simulink model "buck_convertor"  (R2015a)
settings: Solver=ode45  StartTime=0  StopTime=10.5  RelTol=1e-3
libraries: simulink x1, powerlib_meascontrol x1
settings Model: Creator=Dell  LastModifiedBy=Dell

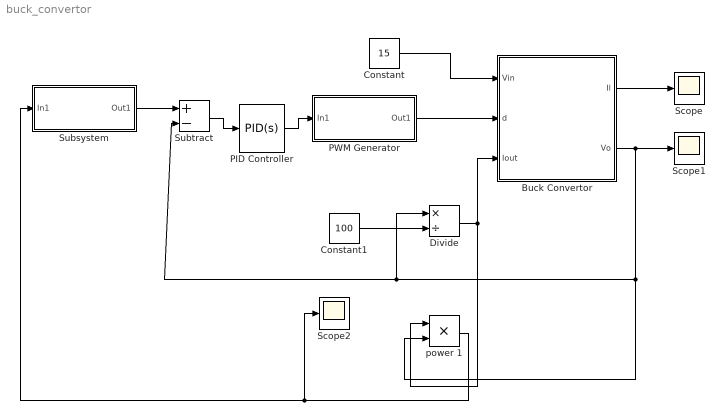
== system buck_convertor ==
  Buck Convertor : Subsystem
  Constant : Constant  Value=15
  Constant1 : Constant  Value=100
  Divide : Product  Inputs=*/
  PID Controller : simulink/Continuous/PID Controller  Controller=PID  TimeDomain=Continuous-time  SampleTime=-1  IntegratorMethod=Forward Euler  FilterMethod=Forward Euler  Form=Parallel  UseFilter=on  ControllerParametersSource=internal  P=1  I=2  D=0  N=1.2  InitialConditionSource=internal  InitialConditionForIntegrator=0  InitialConditionForFilter=0  ExternalReset=none  LimitOutput=off  UpperSaturationLimit=inf  LowerSaturationLimit=-inf  LinearizeAsGain=on  AntiWindupMode=none  Kb=1  TrackingMode=off  Kt=1  PParamMin=[]  PParamMax=[]  IParamMin=[]  IParamMax=[]  DParamMin=[]  DParamMax=[]  NParamMin=[]  NParamMax=[]  KbParamMin=[]  KbParamMax=[]  KtParamMin=[]  KtParamMax=[]  POutMin=[]  POutMax=[]  IOutMin=[]  IOutMax=[]  DOutMin=[]  DOutMax=[]  NOutMin=[]  NOutMax=[]  KbOutMin=[]  KbOutMax=[]  KtOutMin=[]  KtOutMax=[]  IntegratorOutMin=[]  IntegratorOutMax=[]  FilterOutMin=[]  FilterOutMax=[]  SumOutMin=[]  SumOutMax=[]  SumI1OutMin=[]  SumI1OutMax=[]  SumI2OutMin=[]  SumI2OutMax=[]  SumI3OutMin=[]  SumI3OutMax=[]  SumDOutMin=[]  SumDOutMax=[]  SaturationOutMin=[]  SaturationOutMax=[]  IntegratorContinuousStateAttributes=''  IntegratorStateMustResolveToSignalObject=off  IntegratorRTWStateStorageClass=Auto  FilterContinuousStateAttributes=''  FilterStateMustResolveToSignalObject=off  FilterRTWStateStorageClass=Auto  DifferentiatorICPrevScaledInput=0  DifferentiatorOutMin=[]  DifferentiatorOutMax=[]
  PWM Generator : Subsystem
  Scope : Scope
  Scope1 : Scope
      settings: YMin=16.825  YMax=17.025
  Scope2 : Scope
      settings: YMin=16.825  YMax=17.025  SaveName=ScopeData5
  Subsystem : Subsystem
  Subtract : Sum  Inputs=+-
  power 1 : Product  Inputs=**
  wires:
  Subtract/1 -> PID Controller/1
  PID Controller/1 -> PWM Generator/1(In1)
  PWM Generator/1(Out1) -> Buck Convertor/2(d)
  Divide/1 -> Buck Convertor/3(Iout), power 1/1
  Constant1/1 -> Divide/2
  Buck Convertor/1(Il) -> Scope/1
  Buck Convertor/2(Vo) -> Scope1/1, power 1/2, Divide/1, Subtract/2
  Subsystem/1(Out1) -> Subtract/1
  power 1/1 -> Scope2/1, Subsystem/1(In1)
  Constant/1 -> Buck Convertor/1(Vin)

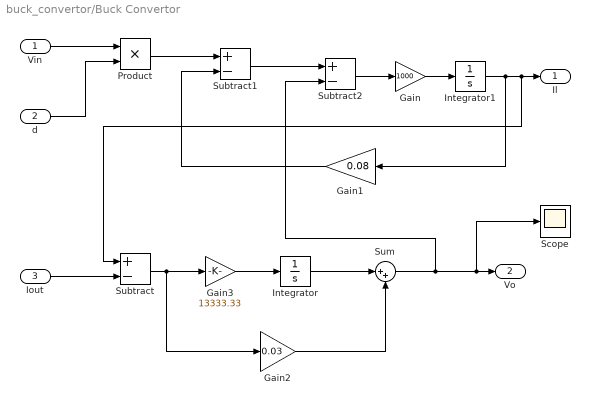
== system buck_convertor/Buck Convertor ==
  Vin : Inport
  d : Inport  Port=2
  Iout : Inport  Port=3
  Gain : Gain  Gain=1000
  Gain1 : Gain  Gain=0.08
  Gain2 : Gain  Gain=0.03
  Gain3 : Gain  Gain=13333.33
  Integrator : Integrator
  Integrator1 : Integrator
  Product : Product
  Scope : Scope
      settings: YMin=16.25  YMax=17.75  SaveName=ScopeData4
  Subtract : Sum  Inputs=+-
  Subtract1 : Sum  Inputs=+-
  Subtract2 : Sum  Inputs=+-
  Sum : Sum  Inputs=|++
  Il : Outport
  Vo : Outport  Port=2
  wires:
  Sum/1 -> Vo/1, Scope/1, Subtract2/2
  Gain2/1 -> Sum/2
  Integrator/1 -> Sum/1
  Gain3/1 -> Integrator/1
  Subtract/1 -> Gain3/1, Gain2/1
  Iout/1 -> Subtract/2
  Gain1/1 -> Subtract1/2
  Integrator1/1 -> Il/1, Subtract/1, Gain1/1
  Gain/1 -> Integrator1/1
  Subtract2/1 -> Gain/1
  Subtract1/1 -> Subtract2/1
  Product/1 -> Subtract1/1
  d/1 -> Product/2
  Vin/1 -> Product/1

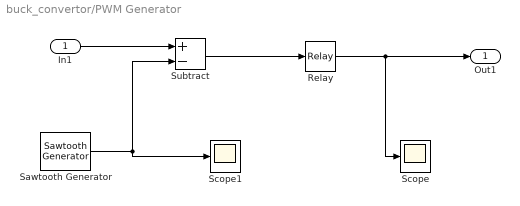
== system buck_convertor/PWM Generator ==
  In1 : Inport
  Relay : Relay  OnSwitchValue=0  OffSwitchValue=0
  Sawtooth Generator : powerlib_meascontrol/Pulse & Signal Generators/Sawtooth Generator  Freq=50000  Phase=180  Ts=0
  Scope : Scope
      settings: SaveName=ScopeData2
  Scope1 : Scope
      settings: SaveName=ScopeData3
  Subtract : Sum  Inputs=+-
  Out1 : Outport
  wires:
  Relay/1 -> Out1/1, Scope/1
  Subtract/1 -> Relay/1
  Sawtooth Generator/1 -> Scope1/1, Subtract/2
  In1/1 -> Subtract/1

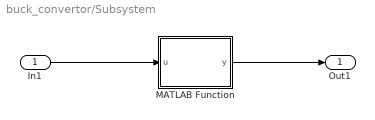
== system buck_convertor/Subsystem ==
  In1 : Inport
  MATLAB Function : MATLAB Function  TreatAsAtomicUnit=on
  Out1 : Outport
  wires:
  In1/1 -> MATLAB Function/1(u)
  MATLAB Function/1(y) -> Out1/1

== matlab function buck_convertor/Subsystem/MATLAB Function ==
  data: u input; y output
function y = fcn(u)
%#codegen
y=u;
